simulink model "ImplementacionRobotPosicionCambiada"  (R2022b)
settings: Solver=ode3  StartTime=0.0  StopTime=100.0  FixedStep=0.01  RelTol=1e-3
undefined symbols (not defined in the file): DiscIntNeverNeededParam
libraries: simulink x9
settings Model: Creator=angy7  LastModifiedBy=angy7

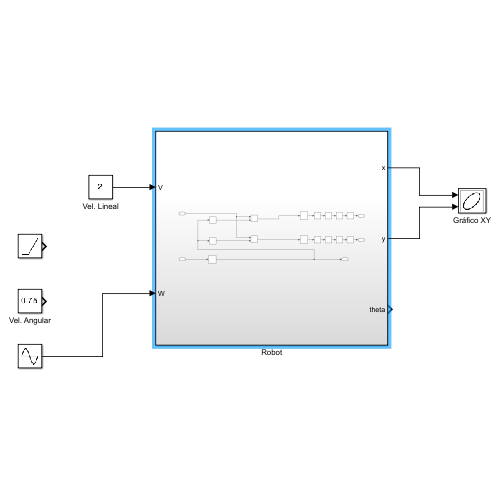
[thumbnail: Simulink's stored preview of the top-level diagram]
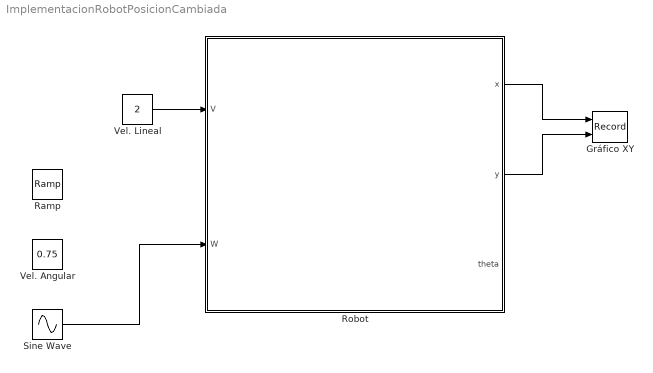
== system ImplementacionRobotPosicionCambiada ==
  Gráfico XY : Record  FileSettingsInternal="{\"entries\":[{\"content\":{\"excelSettings\":{\"content\":{},\"type\":\"Streamout.ExcelSettings\"}},\"type\":\"Streamout.FileSettingStorage\",\"uuid\":\"\"}],\"packageUris\":[\"http:\\/\\/schema.mathworks.com\\/mf0\\/streamout_blocks\\/R2020a\"],\"version\":\"1.0\"}"  Layout=[1 1]  SignalsInternal="{\"entries\":[{\"content\":{\"signals\":[{\"content\":{\"blockPath\":[],\"channel\":[],\"dimensions\":[1],\"domain\":\"\",\"lineColor\":\"#d95319\",\"plots\":[1],\"port\":1,\"sid\":[\"\"],\"signalID\":21300,\"signalName\":\"Robot:1\"},\"type\":\"RecordBlkView.Signal\",\"uuid\":\"\"},{\"content\":{\"blockPath\":[],\"channel\":[],\"dimensions\":[1],\"domain\":\"\",\"lineColor\":\"#d95319\",\"plots\":[],\"port\":2,\"sid\":[\"\"],\"signalID\":21304,\"signalName\":\"Robot:2\"},\"type\":\"RecordBlkView.Signal\",\"uuid\":\"\"}]},\"type\":\"RecordBlkView.InputSignals\",\"uuid\":\"\"}],\"packageUris\":[\"http:\\/\\/schema.mathworks.com\\/mf0\\/streamout_blocks\\/R2020a\"],\"version\":\"1.0\"}"  VisualizationBindings="{\"xyplotplugin\":{\"info\":[{\"series\":[],\"subplotID\":1}]}}"  CompatibilityTag=XY
  Ramp : simulink/Sources/Ramp  slope=1  start=0  InitialOutput=0
  Robot : Subsystem
  Sine Wave : Sin  Amplitude=10  Frequency=10  SampleTime=0
  Vel. Angular : Constant  Value=0.75
  Vel. Lineal : Constant  Value=2
  wires:
  Vel. Lineal/1 -> Robot/1(V)
  Robot/1(x) -> Gráfico XY/1
  Robot/2(y) -> Gráfico XY/2
  Sine Wave/1 -> Robot/2(W)

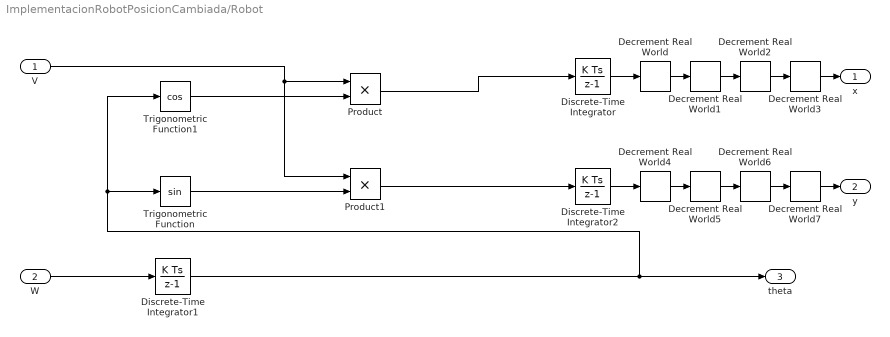
== system ImplementacionRobotPosicionCambiada/Robot ==
  V : Inport
  W : Inport  Port=2
  Decrement Real World{,1..7} (8 alike) : simulink/Additional Math & Discrete/Additional Math: Increment - Decrement/Decrement Real World
  Discrete-Time Integrator : DiscreteIntegrator  SampleTime=-1  ICPrevOutput=DiscIntNeverNeededParam  ICPrevScaledInput=DiscIntNeverNeededParam
  Discrete-Time Integrator1 : DiscreteIntegrator  SampleTime=-1  ICPrevOutput=DiscIntNeverNeededParam  ICPrevScaledInput=DiscIntNeverNeededParam
  Discrete-Time Integrator2 : DiscreteIntegrator  SampleTime=-1  ICPrevOutput=DiscIntNeverNeededParam  ICPrevScaledInput=DiscIntNeverNeededParam
  Product : Product
  Product1 : Product
  Trigonometric Function : Trigonometry
  Trigonometric Function1 : Trigonometry  Operator=cos
  x : Outport
  y : Outport  Port=2
  theta : Outport  Port=3
  wires:
  Trigonometric Function1/1 -> Product/2
  Discrete-Time Integrator2/1 -> Decrement Real World4/1
  Trigonometric Function/1 -> Product1/2
  W/1 -> Discrete-Time Integrator1/1
  Product/1 -> Discrete-Time Integrator/1
  Discrete-Time Integrator1/1 -> Trigonometric Function1/1, Trigonometric Function/1, theta/1
  Product1/1 -> Discrete-Time Integrator2/1
  V/1 -> Product1/1, Product/1
  Discrete-Time Integrator/1 -> Decrement Real World/1
  Decrement Real World/1 -> Decrement Real World1/1
  Decrement Real World1/1 -> Decrement Real World2/1
  Decrement Real World2/1 -> Decrement Real World3/1
  Decrement Real World3/1 -> x/1
  Decrement Real World4/1 -> Decrement Real World5/1
  Decrement Real World5/1 -> Decrement Real World6/1
  Decrement Real World6/1 -> Decrement Real World7/1
  Decrement Real World7/1 -> y/1
